simulink model "Assignment2"  (R2020a)
settings: Solver=FixedStepAuto  StartTime=0.0  StopTime=10.0  FixedStep=1e-3  RelTol=1e-3  EnableMultiTasking=on
settings Model: ExtModeTrigDuration=5  Creator=Ethan  LastModifiedBy=Ethan
settings OptimizationCC: EnhancedBackFolding=on  PassReuseOutputArgsAs=Individual arguments  ZeroExternalMemoryAtStartup=off  ZeroInternalMemoryAtStartup=off  MaxStackSize=64  OptimizeBlockOrder=speed  DifferentSizesBufferReuse=on  OptimizationCustomize=off  EfficientTunableParamExpr=on
settings DebuggingCC: ParameterTunabilityLossMsg=error
settings HardwareCC: ProdBitPerPointer=32  ProdBitPerSizeT=32  ProdBitPerPtrDiffT=32  ProdLargestAtomicInteger=Long  ProdLargestAtomicFloat=Double  ProdWordSize=32  ProdHWDeviceType=ARM Compatible->ARM Cortex
settings SFSimCC: MATLABDynamicMemAlloc=off
settings RTWCC: SystemTargetFile=ert.tlc  HardwareBoard=NXP FRDM-K64F  TemplateMakefile=ert_default_tmf  Toolchain=GNU Tools for ARM Embedded Processors
settings CodeAppCC: ForceParamTrailComments=on  IgnoreCustomStorageClasses=off  OperatorAnnotations=on  SimulinkDataObjDesc=on  SFDataObjDesc=on  InsertBlockDesc=on

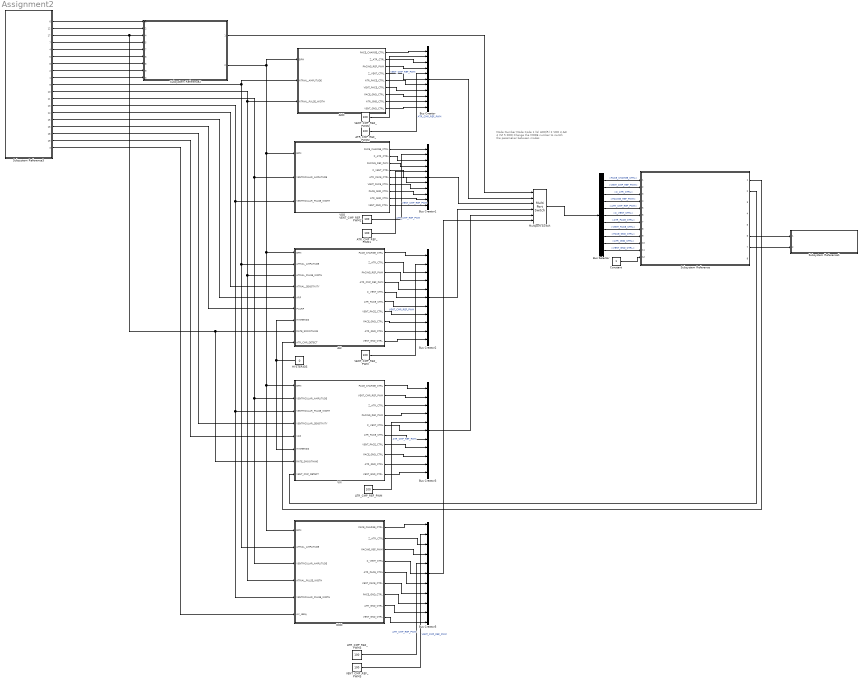
== system Assignment2 ==
  note: Mode Number
      | Mode Code
      |
      | 1 (6)
      | AOO(R)
      |
      | 2
      | VOO
      |
      | 3
      | AAI
      |
      | 4
      | VVI
      |
      | 5
      | DOO
      |
      | Change the MODE number to switch the pacemaker between modes
  AAI : Stateflow chart  TreatAsAtomicUnit=on
      settings: PortSchema="{\"entries\":[{\"content\":{\"sides\":[{\"content\":{\"connectorIds\":[\"In1\",\"In2\",\"In3\",\"In4\",\"In5\",\"In6\",\"In7\",\"In8\",\"In9\"]},\"type\":\"ConnectorPlacement.EquallySpacedRectSide\",\"uuid\":\"b678de6f-9e61-4024-a0aa-5bf6d03f3d0b\"},{\"content\":{\"connectorIds\":[\"Out3\",\"Out8\",\"Out5\",\"Out10\",\"Out9\",\"Out2\",\"Out7\",\"Out4\",\"Out1\",\"Out6\"],\"side\":\"RIGHT\"},\"type\":\"ConnectorPlacement.EquallySpacedRectSide\",\"uuid\":\"4cd0faad-dd9d-4a56-81c5-44f7dd4bee31\"},{\"content\":{\"connectorIds\":[],\"side\":\"TOP\"},\"type\":\"ConnectorPlacement.EquallySpacedRectSide\",\"uuid\":\"a9bc4227-6f84-42c8-b827-a378e14304fe\"},{\"content\":{\"connectorIds\":[],\"side\":\"BOTTOM\"},\"type\":\"ConnectorPlacement.EquallySpacedRectSide\",\"uuid\":\"399184e4-c77f-47b0-89f0-adcbaf01dcf6\"}]},\"type\":\"ConnectorPlacement.EquallySpacedConnector\",\"uuid\":\"ee3b07ee-2423-4f21-89d4-53b7a563517d\"}],\"packageUris\":[\"http://schema.mathworks.com/mf0/Connector/19700101\"],\"version\":\"1.0\"}"
  AOO : Stateflow chart  TreatAsAtomicUnit=on
      settings: PortSchema="{\"entries\":[{\"content\":{\"sides\":[{\"content\":{\"connectorIds\":[\"In1\",\"In2\",\"In3\"]},\"type\":\"ConnectorPlacement.EquallySpacedRectSide\",\"uuid\":\"a22e05d8-b46e-41db-a99f-a3bab389e16c\"},{\"content\":{\"connectorIds\":[\"Out3\",\"Out8\",\"Out5\",\"Out9\",\"Out2\",\"Out7\",\"Out4\",\"Out1\",\"Out6\"],\"side\":\"RIGHT\"},\"type\":\"ConnectorPlacement.EquallySpacedRectSide\",\"uuid\":\"b830ec1d-656a-4b92-afcd-8fda6b31ad8a\"},{\"content\":{\"connectorIds\":[],\"side\":\"TOP\"},\"type\":\"ConnectorPlacement.EquallySpacedRectSide\",\"uuid\":\"956e5d71-b4a8-48ca-aae1-84adff4c1ec1\"}]},\"type\":\"ConnectorPlacement.EquallySpacedConnector\",\"uuid\":\"bd48be11-38ec-46b0-b71c-a53820608697\"}],\"packageUris\":[\"http://schema.mathworks.com/mf0/Connector/19700101\"],\"version\":\"1.0\"}"
  ATR_CMP_REF_PWM{,1..3} (4 alike) : Constant  Value=100
  Bus Creator{,1..3,5} (5 alike) : BusCreator  Inputs=11
  Bus Selector : BusSelector  OutputSignals=PACE_CHARGE_CTRL,VENT_CMP_REF_PWM,Z_ATR_CTRL,PACING_REF_PWM,ATR_CMP_REF_PWM,Z_VENT_CTRL,ATR_PACE_CTRL,VENT_PACE_CTRL,PACE_GND_CTRL,ATR_GND_CTRL,VENT_GND_CTRL
  Constant : Constant
  DOO : Stateflow chart  TreatAsAtomicUnit=on
      settings: PortSchema="{\"entries\":[{\"content\":{\"sides\":[{\"content\":{\"connectorIds\":[\"In2\",\"In6\",\"In5\",\"In3\",\"In4\",\"In1\"]},\"type\":\"ConnectorPlacement.EquallySpacedRectSide\",\"uuid\":\"81f9977c-034e-4b80-9b8d-d1437f78061c\"},{\"content\":{\"connectorIds\":[\"Out5\",\"Out2\",\"Out9\",\"Out8\",\"Out4\",\"Out7\",\"Out1\",\"Out3\",\"Out6\"],\"side\":\"RIGHT\"},\"type\":\"ConnectorPlacement.EquallySpacedRectSide\",\"uuid\":\"78141407-e37e-4be8-94dd-f1101a5ff66d\"},{\"content\":{\"connectorIds\":[],\"side\":\"TOP\"},\"type\":\"ConnectorPlacement.EquallySpacedRectSide\",\"uuid\":\"62f1ae17-2832-4fd3-a4db-2412b9618dd0\"}]},\"type\":\"ConnectorPlacement.EquallySpacedConnector\",\"uuid\":\"b4eedabe-9eda-465b-9a3b-250e05abb6a2\"}],\"packageUris\":[\"http://schema.mathworks.com/mf0/Connector/19700101\"],\"version\":\"1.0\"}"
  HYSTERISIS : Constant  Value=0
  Multiport Switch : MultiPortSwitch  Inputs=5  DiagnosticForDefault=Warning
  Subsystem Reference : Subsystem  ReferencedSubsystem=k64f_subsystem
  Subsystem Reference1 : Subsystem  ReferencedSubsystem=egram_transmitter
  Subsystem Reference2 : Subsystem  ReferencedSubsystem=active_pacing_subsystem
      settings: PortSchema="{\"entries\":[{\"content\":{\"sides\":[{\"content\":{\"connectorIds\":[\"In1\",\"In2\",\"In4\",\"In5\",\"In7\",\"In6\",\"In8\",\"In9\",\"In3\"]},\"type\":\"ConnectorPlacement.EquallySpacedRectSide\",\"uuid\":\"81983024-f78a-47c3-92f3-f29553261ea8\"},{\"content\":{\"connectorIds\":[\"Out1\",\"Out2\"],\"side\":\"RIGHT\"},\"type\":\"ConnectorPlacement.EquallySpacedRectSide\",\"uuid\":\"9875b86f-c0b3-4704-98d1-70e4bf13acc8\"},{\"content\":{\"connectorIds\":[],\"side\":\"TOP\"},\"type\":\"ConnectorPlacement.EquallySpacedRectSide\",\"uuid\":\"fa24a894-4ee7-4a9e-af4e-dad9c3d2769f\"}]},\"type\":\"ConnectorPlacement.EquallySpacedConnector\",\"uuid\":\"2c33192a-fb1f-4370-903d-51784514e1cc\"}],\"packageUris\":[\"http://schema.mathworks.com/mf0/Connector/19700101\"],\"version\":\"1.0\"}"
  Subsystem Reference3 : Subsystem  ReferencedSubsystem=serial_input_subsystem
      settings: PortSchema="{\"entries\":[{\"content\":{\"sides\":[{\"content\":{\"connectorIds\":[]},\"type\":\"ConnectorPlacement.EquallySpacedRectSide\",\"uuid\":\"ea718484-7b85-4066-a394-acd8a1350ae7\"},{\"content\":{\"connectorIds\":[\"Out6\",\"Out12\",\"Out17\",\"Out7\",\"Out4\",\"Out5\",\"Out8\",\"Out2\",\"Out1\",\"Out9\",\"Out10\",\"Out11\",\"Out13\",\"Out14\",\"Out15\",\"Out16\",\"Out18\",\"Out19\",\"Out3\"],\"side\":\"RIGHT\"},\"type\":\"ConnectorPlacement.EquallySpacedRectSide\",\"uuid\":\"0c0c1125-8bcf-4fa8-bc6a-7859181eb93b\"},{\"content\":{\"connectorIds\":[],\"side\":\"TOP\"},\"type\":\"ConnectorPlacement.EquallySpacedRectSide\",\"uuid\":\"1a473457-4ed6-4a33-897e-c1d07c0c36a8\"}]},\"type\":\"ConnectorPlacement.EquallySpacedConnector\",\"uuid\":\"8727b5bd-ade5-46de-83df-763247b1aa59\"}],\"packageUris\":[\"http://schema.mathworks.com/mf0/Connector/19700101\"],\"version\":\"1.0\"}"
  VENT_CMP_REF_PWM{,1..3} (4 alike) : Constant  Value=100
  VOO : Stateflow chart  TreatAsAtomicUnit=on
      settings: PortSchema="{\"entries\":[{\"content\":{\"sides\":[{\"content\":{\"connectorIds\":[\"In1\",\"In2\",\"In3\"]},\"type\":\"ConnectorPlacement.EquallySpacedRectSide\",\"uuid\":\"a22e05d8-b46e-41db-a99f-a3bab389e16c\"},{\"content\":{\"connectorIds\":[\"Out3\",\"Out8\",\"Out5\",\"Out9\",\"Out2\",\"Out7\",\"Out4\",\"Out1\",\"Out6\"],\"side\":\"RIGHT\"},\"type\":\"ConnectorPlacement.EquallySpacedRectSide\",\"uuid\":\"b830ec1d-656a-4b92-afcd-8fda6b31ad8a\"},{\"content\":{\"connectorIds\":[],\"side\":\"TOP\"},\"type\":\"ConnectorPlacement.EquallySpacedRectSide\",\"uuid\":\"956e5d71-b4a8-48ca-aae1-84adff4c1ec1\"}]},\"type\":\"ConnectorPlacement.EquallySpacedConnector\",\"uuid\":\"bd48be11-38ec-46b0-b71c-a53820608697\"}],\"packageUris\":[\"http://schema.mathworks.com/mf0/Connector/19700101\"],\"version\":\"1.0\"}"
  VVI : Stateflow chart  TreatAsAtomicUnit=on
      settings: PortSchema="{\"entries\":[{\"content\":{\"sides\":[{\"content\":{\"connectorIds\":[\"In1\",\"In2\",\"In3\",\"In4\",\"In5\",\"In6\",\"In7\",\"In8\"]},\"type\":\"ConnectorPlacement.EquallySpacedRectSide\",\"uuid\":\"b678de6f-9e61-4024-a0aa-5bf6d03f3d0b\"},{\"content\":{\"connectorIds\":[\"Out3\",\"Out10\",\"Out8\",\"Out5\",\"Out9\",\"Out2\",\"Out7\",\"Out4\",\"Out1\",\"Out6\"],\"side\":\"RIGHT\"},\"type\":\"ConnectorPlacement.EquallySpacedRectSide\",\"uuid\":\"4cd0faad-dd9d-4a56-81c5-44f7dd4bee31\"},{\"content\":{\"connectorIds\":[],\"side\":\"TOP\"},\"type\":\"ConnectorPlacement.EquallySpacedRectSide\",\"uuid\":\"a9bc4227-6f84-42c8-b827-a378e14304fe\"},{\"content\":{\"connectorIds\":[],\"side\":\"BOTTOM\"},\"type\":\"ConnectorPlacement.EquallySpacedRectSide\",\"uuid\":\"d9bc86ca-c62d-429e-b855-d0c137c2bc24\"}]},\"type\":\"ConnectorPlacement.EquallySpacedConnector\",\"uuid\":\"ee3b07ee-2423-4f21-89d4-53b7a563517d\"}],\"packageUris\":[\"http://schema.mathworks.com/mf0/Connector/19700101\"],\"version\":\"1.0\"}"
  wires:
  Bus Selector/1 -> Subsystem Reference/1  "<PACE_CHARGE_CTRL>"
  VENT_CMP_REF_PWM1/1 -> Bus Creator1/2  "VENT_CMP_REF_PWM"
  AOO/7(VENT_PACE_CTRL) -> Bus Creator/8
  AAI/7(VENT_PACE_CTRL) -> Bus Creator2/8
  HYSTERISIS/1 -> AAI/7(HYSTERISIS), VVI/6(HYSTERISIS)
  AAI/9(Z_VENT_CTRL) -> Bus Creator2/6
  Multiport Switch/1 -> Bus Selector/1
  ATR_CMP_REF_PWM2/1 -> Bus Creator/5  "ATR_CMP_REF_PWM"
  VVI/7(VENT_PACE_CTRL) -> Bus Creator3/8
  AAI/8(Z_ATR_CTRL) -> Bus Creator2/3
  Bus Selector/11 -> Subsystem Reference/11  "<VENT_GND_CTRL>"
  AOO/5(PACING_REF_PWM) -> Bus Creator/4
  Bus Selector/3 -> Subsystem Reference/3  "<Z_ATR_CTRL>"
  VOO/5(PACING_REF_PWM) -> Bus Creator1/4
  Bus Selector/4 -> Subsystem Reference/4  "<PACING_REF_PWM>"
  ATR_CMP_REF_PWM/1 -> Bus Creator3/5  "ATR_CMP_REF_PWM"
  AAI/3(PACE_CHARGE_CTRL) -> Bus Creator2/1
  Bus Creator2/1 -> Multiport Switch/4
  Bus Selector/6 -> Subsystem Reference/6  "<Z_VENT_CTRL>"
  VENT_CMP_REF_PWM/1 -> Bus Creator2/2  "VENT_CMP_REF_PWM"
  VVI/4(PACE_GND_CTRL) -> Bus Creator3/9
  AAI/2(ATR_PACE_CTRL) -> Bus Creator2/7
  Bus Selector/9 -> Subsystem Reference/9  "<PACE_GND_CTRL>"
  VVI/9(Z_VENT_CTRL) -> Bus Creator3/6
  VVI/5(PACING_REF_PWM) -> Bus Creator3/4
  Constant/1 -> Subsystem Reference/12
  Subsystem Reference/2 -> VVI/8(VENT_CMP_DETECT)
  AAI/6(VENT_GND_CTRL) -> Bus Creator2/11
  AAI/10(ATR_CMP_REF_PWM) -> Bus Creator2/5
  VVI/3(PACE_CHARGE_CTRL) -> Bus Creator3/1
  VOO/2(ATR_PACE_CTRL) -> Bus Creator1/7
  Bus Selector/7 -> Subsystem Reference/7  "<ATR_PACE_CTRL>"
  VVI/6(VENT_GND_CTRL) -> Bus Creator3/11
  Bus Selector/10 -> Subsystem Reference/10  "<ATR_GND_CTRL>"
  AOO/9(Z_VENT_CTRL) -> Bus Creator/6
  Bus Selector/5 -> Subsystem Reference/5  "<ATR_CMP_REF_PWM>"
  VVI/2(ATR_PACE_CTRL) -> Bus Creator3/7
  Bus Creator/1 -> Multiport Switch/2
  VVI/10(VENT_CMP_REF_PWM) -> Bus Creator3/2
  VVI/1(ATR_GND_CTRL) -> Bus Creator3/10
  Bus Creator1/1 -> Multiport Switch/3
  VOO/1(ATR_GND_CTRL) -> Bus Creator1/10
  AOO/8(Z_ATR_CTRL) -> Bus Creator/3
  VOO/6(VENT_GND_CTRL) -> Bus Creator1/11
  AOO/6(VENT_GND_CTRL) -> Bus Creator/11
  AOO/1(ATR_GND_CTRL) -> Bus Creator/10
  VOO/8(Z_ATR_CTRL) -> Bus Creator1/3
  AAI/1(ATR_GND_CTRL) -> Bus Creator2/10
  Subsystem Reference/1 -> AAI/9(ATR_CMP_DETECT)
  ATR_CMP_REF_PWM1/1 -> Bus Creator1/5  "ATR_CMP_REF_PWM"
  VENT_CMP_REF_PWM2/1 -> Bus Creator/2  "VENT_CMP_REF_PWM"
  AOO/3(PACE_CHARGE_CTRL) -> Bus Creator/1
  VVI/8(Z_ATR_CTRL) -> Bus Creator3/3
  AOO/4(PACE_GND_CTRL) -> Bus Creator/9
  AOO/2(ATR_PACE_CTRL) -> Bus Creator/7
  VOO/3(PACE_CHARGE_CTRL) -> Bus Creator1/1
  VOO/4(PACE_GND_CTRL) -> Bus Creator1/9
  Bus Creator3/1 -> Multiport Switch/5
  VOO/7(VENT_PACE_CTRL) -> Bus Creator1/8
  AAI/5(PACING_REF_PWM) -> Bus Creator2/4
  Bus Selector/8 -> Subsystem Reference/8  "<VENT_PACE_CTRL>"
  AAI/4(PACE_GND_CTRL) -> Bus Creator2/9
  Bus Selector/2 -> Subsystem Reference/2  "<VENT_CMP_REF_PWM>"
  VOO/9(Z_VENT_CTRL) -> Bus Creator1/6
  DOO/1(PACE_GND_CTRL) -> Bus Creator5/9
  DOO/6(VENT_GND_CTRL) -> Bus Creator5/11
  DOO/3(ATR_GND_CTRL) -> Bus Creator5/10
  DOO/7(VENT_PACE_CTRL) -> Bus Creator5/8
  DOO/4(ATR_PACE_CTRL) -> Bus Creator5/7
  DOO/5(PACE_CHARGE_CTRL) -> Bus Creator5/1
  DOO/2(Z_ATR_CTRL) -> Bus Creator5/3
  DOO/9(PACING_REF_PWM) -> Bus Creator5/4
  VENT_CMP_REF_PWM3/1 -> Bus Creator5/2  "VENT_CMP_REF_PWM"
  DOO/8(Z_VENT_CTRL) -> Bus Creator5/6
  ATR_CMP_REF_PWM3/1 -> Bus Creator5/5  "ATR_CMP_REF_PWM"
  Bus Creator5/1 -> Multiport Switch/6
  Subsystem Reference/6 -> Subsystem Reference1/1
  Subsystem Reference/7 -> Subsystem Reference1/2
  Subsystem Reference3/6 -> Subsystem Reference2/1
  Subsystem Reference3/12 -> Subsystem Reference2/2
  Subsystem Reference3/17 -> VVI/7(RATE_SMOOTHING), AAI/8(RATE_SMOOTHING), Subsystem Reference2/4
  Subsystem Reference3/7 -> Subsystem Reference2/5
  Subsystem Reference3/4 -> Subsystem Reference2/7
  Subsystem Reference3/8 -> Subsystem Reference2/8
  Subsystem Reference3/5 -> Subsystem Reference2/6
  Subsystem Reference3/11 -> DOO/5(VENTRICULAR_AMPLITUDE), VVI/2(VENTRICULAR_AMPLITUDE), VOO/2(VENTRICULAR_AMPLITUDE)
  Subsystem Reference3/10 -> DOO/3(ATRIAL_PULSE_WIDTH), AAI/3(ATRIAL_PULSE_WIDTH), AOO/3(ATRIAL_PULSE_WIDTH)
  Subsystem Reference3/9 -> AOO/2(ATRIAL_AMPLITUDE), DOO/6(ATRIAL_AMPLITUDE), AAI/2(ATRIAL_AMPLITUDE)
  Subsystem Reference3/13 -> DOO/4(VENTRICULAR_PULSE_WIDTH), VVI/3(VENTRICULAR_PULSE_WIDTH), VOO/3(VENTRICULAR_PULSE_WIDTH)
  Subsystem Reference3/14 -> AAI/4(ATRIAL_SENSITIVITY)
  Subsystem Reference3/2 -> Subsystem Reference2/9
  Subsystem Reference3/15 -> AAI/5(ARP)
  Subsystem Reference3/16 -> AAI/6(PVARP)
  Subsystem Reference3/18 -> VVI/4(VENTRICULAR_SENSITIVITY)
  Subsystem Reference3/19 -> VVI/5(VRP)
  Subsystem Reference3/3 -> DOO/1(AV_delay)
  Subsystem Reference2/2 -> AOO/1(BPM), VOO/1(BPM), VVI/1(BPM), DOO/2(BPM), AAI/1(BPM)
  Subsystem Reference2/1 -> Multiport Switch/1
  Subsystem Reference3/1 -> Subsystem Reference2/3

== stateflow chart Assignment2/AOO ==
  note: AOO mode paces the atrium at a constant rate regardless of the natural heartbeat
  state PULSE_ATR
    entry:
    PACE_CHARGE_CTRL = 0;
    PACE_GND_CTRL = 1;
    VENT_GND_CTRL = 0;
    VENT_PACE_CTRL = 0;
    Z_ATR_CTRL = 0;
    Z_VENT_CTRL = 0;
    ATR_GND_CTRL = 0;
    ATR_PACE_CTRL = 1;
  state CHARGE
    entry:
    ATR_PACE_CTRL = 0;
    VENT_PACE_CTRL = 0;
    PACING_REF_PWM = ATRIAL_AMPLITUDE;
    PACE_CHARGE_CTRL = 1;
  state DISCHARGE
    entry:
    PACE_GND_CTRL = 1;
    VENT_PACE_CTRL = 0;
    Z_ATR_CTRL = 0;
    Z_VENT_CTRL = 0;
    ATR_PACE_CTRL = 0;
    ATR_GND_CTRL = 0;
    VENT_GND_CTRL = 1;
  (default) -> CHARGE
  CHARGE -> PULSE_ATR : after(60/BPM,sec)
  DISCHARGE -> CHARGE
  PULSE_ATR -> DISCHARGE : after(ATRIAL_PULSE_WIDTH, msec)
  data: ATR_GND_CTRL output; ATR_PACE_CTRL output; PACE_CHARGE_CTRL output; PACE_GND_CTRL output; PACING_REF_PWM output; VENT_GND_CTRL output; VENT_PACE_CTRL output; Z_ATR_CTRL output; Z_VENT_CTRL output; BPM input; ATRIAL_AMPLITUDE input; ATRIAL_PULSE_WIDTH input

== stateflow chart Assignment2/VVI ==
  note: VVI will only pace the ventricle if the natural heartbeat drops below that of the defined lower limit
  state hold
    entry:
  note: skip pulse if natural heart beat is detected
  state PULSE_SET_NATURAL
    entry:
    last_pulse_natural = true;
  state PULSE_SET_ARTIFICIAL
    entry:
    last_pulse_natural = false;
  state PULSE_VENT
    entry:
    PACE_CHARGE_CTRL = 0;
    VENT_GND_CTRL = 0;
    VENT_PACE_CTRL = 1;
  state CHARGE
    entry:
    VENT_PACE_CTRL = 0;
    PACE_CHARGE_CTRL = 1;
  state INIT
    entry:
    VENT_CMP_REF_PWM = VENTRICULAR_SENSITIVITY;
    PACING_REF_PWM = VENTRICULAR_AMPLITUDE;
    ATR_GND_CTRL = 0;
    ATR_PACE_CTRL = 0;
    Z_ATR_CTRL = 0;
    Z_VENT_CTRL = 0;
    PACE_GND_CTRL = 1;
    last_pulse_natural = false;
  state DISCHARGE
    entry:
    VENT_PACE_CTRL = 0;
    VENT_GND_CTRL = 1;
  hold -> PULSE_SET_ARTIFICIAL [order 2] : after(60000/uint16(BPM)-VENTRICULAR_PULSE_WIDTH-VRP, msec)[ last_pulse_natural == false || HYSTERISIS == 0]
  CHARGE -> hold : after(VRP, msec)
  hold -> PULSE_SET_ARTIFICIAL [order 3] : after(60000/(uint16(BPM)-HYSTERISIS)-VRP, msec)[ last_pulse_natural == true && HYSTERISIS > 0]
  hold -> PULSE_SET_NATURAL [order 1] : [VENT_CMP_DETECT == 1]
  PULSE_SET_ARTIFICIAL -> PULSE_VENT
  PULSE_SET_NATURAL -> CHARGE
  INIT -> CHARGE
  PULSE_VENT -> DISCHARGE : after(VENTRICULAR_PULSE_WIDTH, msec)
  (default) -> INIT
  DISCHARGE -> INIT
  data: ATR_GND_CTRL output; ATR_PACE_CTRL output; PACE_CHARGE_CTRL output; PACE_GND_CTRL output; PACING_REF_PWM output; VENT_GND_CTRL output; VENT_PACE_CTRL output; Z_ATR_CTRL output; Z_VENT_CTRL output; BPM input; VENTRICULAR_AMPLITUDE input; VENTRICULAR_PULSE_WIDTH input; VENTRICULAR_SENSITIVITY input; VRP input; HYSTERISIS input; RATE_SMOOTHING input; VENT_CMP_REF_PWM output; VENT_CMP_DETECT input; last_pulse_natural local

== stateflow chart Assignment2/DOO ==
  note: DOO mode paces the atrium then ventricle at a constant rate regardless of the natural heartbeat
  state PULSE_ATR
    entry:
    PACE_CHARGE_CTRL = 0;
    PACE_GND_CTRL = 1;
    VENT_GND_CTRL = 0;
    VENT_PACE_CTRL = 0;
    Z_ATR_CTRL = 0;
    Z_VENT_CTRL = 0;
    ATR_GND_CTRL = 0;
    ATR_PACE_CTRL = 1;
  state CHARGE
    entry:
    ATR_PACE_CTRL = 0;
    VENT_PACE_CTRL = 0;
    PACING_REF_PWM = ATRIAL_AMPLITUDE;
    PACE_CHARGE_CTRL = 1;
  state DISCHARGE
    entry:
    PACE_GND_CTRL = 1;
    VENT_PACE_CTRL = 0;
    Z_ATR_CTRL = 0;
    Z_VENT_CTRL = 0;
    ATR_PACE_CTRL = 0;
    ATR_GND_CTRL = 1;
    VENT_GND_CTRL = 0;
  state CHARGE1
    entry:
    ATR_PACE_CTRL = 0;
    VENT_PACE_CTRL = 0;
    PACING_REF_PWM = VENTRICULAR_AMPLITUDE;
    PACE_CHARGE_CTRL = 1;
  state PULSE_VENT
    entry:
    PACE_CHARGE_CTRL = 0;
    PACE_GND_CTRL = 1;
    ATR_PACE_CTRL = 0;
    ATR_GND_CTRL = 0;
    Z_ATR_CTRL = 0;
    Z_VENT_CTRL = 0;
    VENT_GND_CTRL = 0;
    VENT_PACE_CTRL = 1;
  state DISCHARGE1
    entry:
    PACE_GND_CTRL = 1;
    VENT_PACE_CTRL = 0;
    Z_ATR_CTRL = 0;
    Z_VENT_CTRL = 0;
    ATR_PACE_CTRL = 0;
    ATR_GND_CTRL = 0;
    VENT_GND_CTRL = 1;
  (default) -> CHARGE
  CHARGE -> PULSE_ATR : after(60/uint16(BPM)*1000 - AV_delay, msec)
  DISCHARGE1 -> CHARGE
  PULSE_ATR -> DISCHARGE : after(ATRIAL_PULSE_WIDTH, msec)
  DISCHARGE -> CHARGE1
  CHARGE1 -> PULSE_VENT : after(AV_delay+ATRIAL_PULSE_WIDTH,msec)
  PULSE_VENT -> DISCHARGE1 : after(VENTRICULAR_PULSE_WIDTH, msec)
  data: PACE_GND_CTRL output; Z_ATR_CTRL output; AV_delay input; BPM input; ATR_GND_CTRL output; ATR_PACE_CTRL output; PACE_CHARGE_CTRL output; VENT_GND_CTRL output; VENT_PACE_CTRL output; Z_VENT_CTRL output; ATRIAL_PULSE_WIDTH input; VENTRICULAR_PULSE_WIDTH input; VENTRICULAR_AMPLITUDE input; ATRIAL_AMPLITUDE input; PACING_REF_PWM output

== stateflow chart Assignment2/VOO ==
  note: VOO mode paces the ventricle at a constant rate regardless of the natural heartbeat
  state PULSE_VENT
    entry:
    PACE_CHARGE_CTRL = 0;
    PACE_GND_CTRL = 1;
    ATR_PACE_CTRL = 0;
    ATR_GND_CTRL = 0;
    Z_ATR_CTRL = 0;
    Z_VENT_CTRL = 0;
    VENT_GND_CTRL = 0;
    VENT_PACE_CTRL = 1;
  state CHARGE
    entry:
    ATR_PACE_CTRL = 0;
    VENT_PACE_CTRL = 0;
    PACING_REF_PWM = VENTRICULAR_AMPLITUDE;
    PACE_CHARGE_CTRL = 1;
  state DISCHARGE
    entry:
    PACE_GND_CTRL = 1;
    VENT_PACE_CTRL = 0;
    Z_ATR_CTRL = 0;
    Z_VENT_CTRL = 0;
    ATR_PACE_CTRL = 0;
    ATR_GND_CTRL = 0;
    VENT_GND_CTRL = 1;
  (default) -> CHARGE
  CHARGE -> PULSE_VENT : after(60/BPM,sec)
  DISCHARGE -> CHARGE
  PULSE_VENT -> DISCHARGE : after(VENTRICULAR_PULSE_WIDTH, msec)
  data: ATR_GND_CTRL output; ATR_PACE_CTRL output; PACE_CHARGE_CTRL output; PACE_GND_CTRL output; PACING_REF_PWM output; VENT_GND_CTRL output; VENT_PACE_CTRL output; Z_ATR_CTRL output; Z_VENT_CTRL output; BPM input; VENTRICULAR_AMPLITUDE input; VENTRICULAR_PULSE_WIDTH input

== stateflow chart Assignment2/AAI ==
  note: AAI will only pace the atrium if the natural heartbeat drops below that of the defined lower limit
  state hold
    entry:
  note: skip pulse if natural heart beat is detected
  state PULSE_SET_NATURAL
    entry:
    last_pulse_natural = true;
  state PULSE_SET_ARTIFICIAL
    entry:
    last_pulse_natural = false;
  state PULSE_ATR
    entry:
    PACE_CHARGE_CTRL = 0;
    ATR_GND_CTRL = 0;
    ATR_PACE_CTRL = 1;
  state CHARGE
    entry:
    ATR_PACE_CTRL = 0;
    PACE_CHARGE_CTRL = 1;
  state INIT
    entry:
    ATR_CMP_REF_PWM = ATRIAL_SENSITIVITY;
    PACING_REF_PWM = ATRIAL_AMPLITUDE;
    VENT_GND_CTRL = 0;
    VENT_PACE_CTRL = 0;
    Z_ATR_CTRL = 0;
    Z_VENT_CTRL = 0;
    PACE_GND_CTRL = 1;
    last_pulse_natural = false;
  state DISCHARGE
    entry:
    ATR_PACE_CTRL = 0;
    ATR_GND_CTRL = 1;
  hold -> PULSE_SET_ARTIFICIAL [order 2] : after(60000/uint16(BPM)-ARP, msec)[ last_pulse_natural == false || HYSTERISIS == 0]
  CHARGE -> hold : after(ARP, msec)
  hold -> PULSE_SET_ARTIFICIAL [order 3] : after(60000/(uint16(BPM)-HYSTERISIS)-ARP, msec)[ last_pulse_natural == true && HYSTERISIS > 0]
  hold -> PULSE_SET_NATURAL [order 1] : [ATR_CMP_DETECT == 1]
  PULSE_SET_ARTIFICIAL -> PULSE_ATR
  PULSE_SET_NATURAL -> CHARGE
  INIT -> CHARGE
  PULSE_ATR -> DISCHARGE : after(ATRIAL_PULSE_WIDTH, msec)
  (default) -> INIT
  DISCHARGE -> INIT
  data: ATR_GND_CTRL output; ATR_PACE_CTRL output; PACE_CHARGE_CTRL output; PACE_GND_CTRL output; PACING_REF_PWM output; VENT_GND_CTRL output; VENT_PACE_CTRL output; Z_ATR_CTRL output; Z_VENT_CTRL output; BPM input; ATRIAL_AMPLITUDE input; ATRIAL_PULSE_WIDTH input; ATRIAL_SENSITIVITY input; ARP input; PVARP input; HYSTERISIS input; RATE_SMOOTHING input; last_pulse_natural local; ATR_CMP_DETECT input; ATR_CMP_REF_PWM output
